simulink subsystem "OneActuatorRWD"  (R2024a)
settings: Solver=VariableStepAuto  StartTime=0.0  StopTime=10.0  RelTol=1e-3
settings Model: Creator=The MathWorks, Inc.  LastModifiedBy=The MathWorks, Inc.
settings RTWCC: GPUComputeCapability=3.5

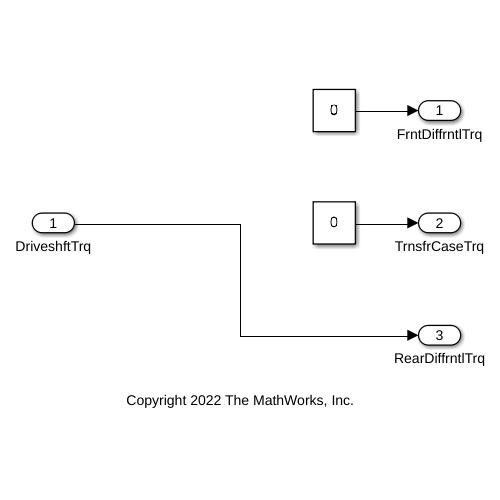
[thumbnail: Simulink's stored preview of the top-level diagram]
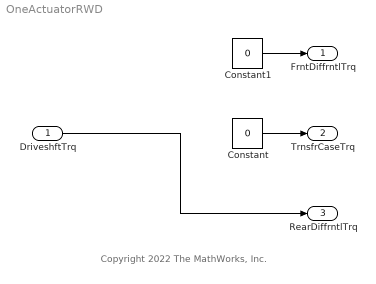
== system OneActuatorRWD ==
  note: Copyright 2022 The MathWorks, Inc.
  DriveshftTrq : Inport
  Constant : Constant  Value=0  SampleTime=-1
  Constant1 : Constant  Value=0  SampleTime=-1
  FrntDiffrntlTrq : Outport
  TrnsfrCaseTrq : Outport  Port=2
  RearDiffrntlTrq : Outport  Port=3
  wires:
  Constant/1 -> TrnsfrCaseTrq/1
  DriveshftTrq/1 -> RearDiffrntlTrq/1
  Constant1/1 -> FrntDiffrntlTrq/1
